simulink model "DRISHTI_District_Telemedicine_Simulation"  (R2026a)
settings: Solver=FixedStepDiscrete  StopTime=1  FixedStep=1
undefined symbols (not defined in the file or in its folder): DRISHTI_aiProcessingSeconds, DRISHTI_aiUnits, DRISHTI_bandwidthMbps, DRISHTI_imageSizeMB, DRISHTI_patientsPerHour, DRISHTI_referableRate, DRISHTI_reviewers, DRISHTI_reviewSeconds

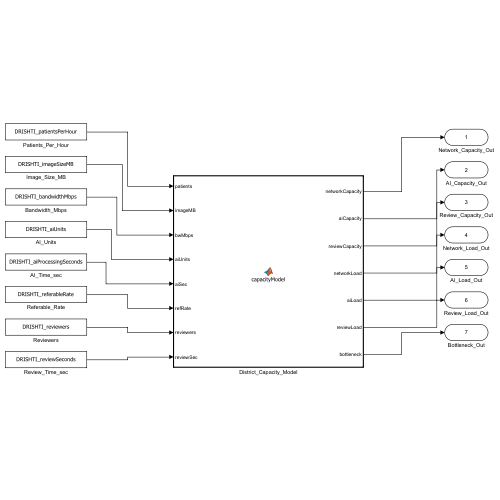
[thumbnail: Simulink's stored preview of the top-level diagram]
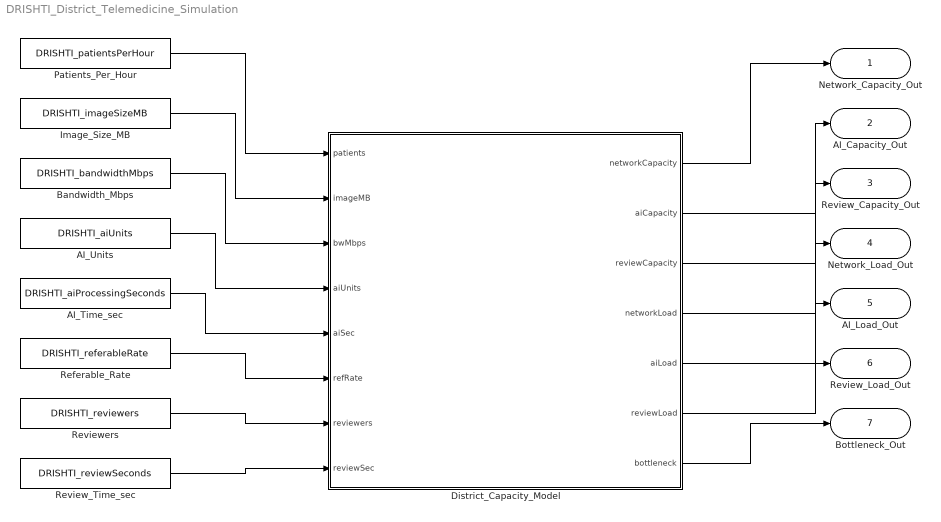
== system DRISHTI_District_Telemedicine_Simulation ==
  AI_Time_sec : Constant  Value=DRISHTI_aiProcessingSeconds
  AI_Units : Constant  Value=DRISHTI_aiUnits
  Bandwidth_Mbps : Constant  Value=DRISHTI_bandwidthMbps
  District_Capacity_Model : MATLAB Function  TreatAsAtomicUnit=on
  Image_Size_MB : Constant  Value=DRISHTI_imageSizeMB
  Patients_Per_Hour : Constant  Value=DRISHTI_patientsPerHour
  Referable_Rate : Constant  Value=DRISHTI_referableRate
  Review_Time_sec : Constant  Value=DRISHTI_reviewSeconds
  Reviewers : Constant  Value=DRISHTI_reviewers
  Network_Capacity_Out : Outport
  AI_Capacity_Out : Outport  Port=2
  Review_Capacity_Out : Outport  Port=3
  Network_Load_Out : Outport  Port=4
  AI_Load_Out : Outport  Port=5
  Review_Load_Out : Outport  Port=6
  Bottleneck_Out : Outport  Port=7
  wires:
  Patients_Per_Hour/1 -> District_Capacity_Model/1(patients)
  Image_Size_MB/1 -> District_Capacity_Model/2(imageMB)
  Bandwidth_Mbps/1 -> District_Capacity_Model/3(bwMbps)
  AI_Units/1 -> District_Capacity_Model/4(aiUnits)
  AI_Time_sec/1 -> District_Capacity_Model/5(aiSec)
  Referable_Rate/1 -> District_Capacity_Model/6(refRate)
  Reviewers/1 -> District_Capacity_Model/7(reviewers)
  Review_Time_sec/1 -> District_Capacity_Model/8(reviewSec)
  District_Capacity_Model/1(networkCapacity) -> Network_Capacity_Out/1
  District_Capacity_Model/2(aiCapacity) -> AI_Capacity_Out/1
  District_Capacity_Model/3(reviewCapacity) -> Review_Capacity_Out/1
  District_Capacity_Model/4(networkLoad) -> Network_Load_Out/1
  District_Capacity_Model/5(aiLoad) -> AI_Load_Out/1
  District_Capacity_Model/6(reviewLoad) -> Review_Load_Out/1
  District_Capacity_Model/7(bottleneck) -> Bottleneck_Out/1

== matlab function DRISHTI_District_Telemedicine_Simulation/District_Capacity_Model ==
  data: patients input; networkCapacity output; imageMB input; bwMbps input; aiUnits input; aiSec input; refRate input; reviewers input; reviewSec input; aiCapacity output; reviewCapacity output; networkLoad output; aiLoad output; reviewLoad output; bottleneck output
function [networkCapacity,aiCapacity,reviewCapacity,networkLoad,aiLoad,reviewLoad,bottleneck] = capacityModel(patients,imageMB,bwMbps,aiUnits,aiSec,refRate,reviewers,reviewSec)
networkCapacity = (bwMbps*3600)/(8*imageMB);
aiCapacity = aiUnits*(3600/aiSec);
reviewCapacity = reviewers*(3600/reviewSec);
networkLoad = patients;
aiLoad = patients;
reviewLoad = patients*refRate;
if networkLoad > networkCapacity
    bottleneck = 1;
elseif aiLoad > aiCapacity
    bottleneck = 2;
elseif reviewLoad > reviewCapacity
    bottleneck = 3;
else
    bottleneck = 0;
end
end
